simulink model "sampleModel1963_1"  (R2023a)
settings: Solver=VariableStepAuto  StartTime=0.0  StopTime=10.0  RelTol=1e-3
libraries: hdlsllib x5
settings Model: Creator=user1  LastModifiedBy=user1

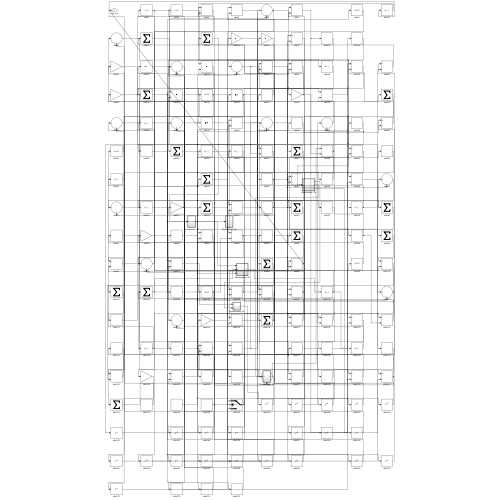
[thumbnail: Simulink's stored preview of the top-level diagram]
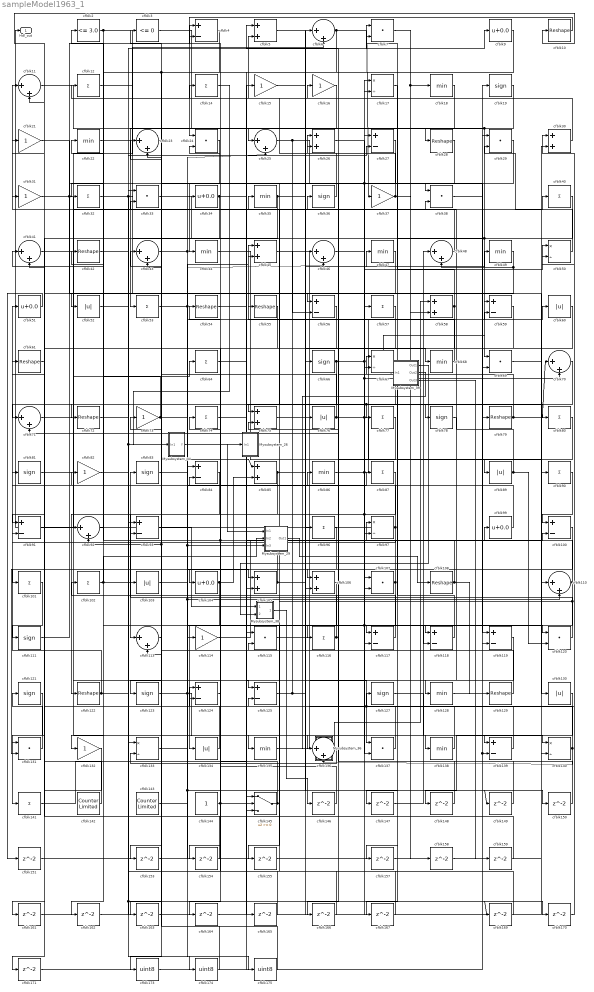
== system sampleModel1963_1 ==
  Mysubsystem_26 : Subsystem  TreatAsAtomicUnit=on  RTWFcnName=Mysubsystem_26
      settings: RTWFcnNameOpts=User specified  RTWFileNameOpts=Use function name
  Mysubsystem_29 : Subsystem  TreatAsAtomicUnit=on  RTWFcnName=Mysubsystem_29
      settings: RTWFcnNameOpts=User specified  RTWFileNameOpts=Use function name
  Mysubsystem_34 : Subsystem  TreatAsAtomicUnit=on  RTWFcnName=Mysubsystem_34
      settings: RTWFcnNameOpts=User specified  RTWFileNameOpts=Use function name
  Mysubsystem_36 : Subsystem  TreatAsAtomicUnit=on  RTWFcnName=Mysubsystem_36
      settings: RTWFcnNameOpts=User specified  RTWFileNameOpts=Use function name
  Mysubsystem_38 : Subsystem  TreatAsAtomicUnit=on  RTWFcnName=Mysubsystem_38
      settings: RTWFcnNameOpts=User specified  RTWFileNameOpts=Use function name
  Mysubsystem_39 : Subsystem  TreatAsAtomicUnit=on  RTWFcnName=Mysubsystem_39
      settings: RTWFcnNameOpts=User specified  RTWFileNameOpts=Use function name
  cfblk{10,28,42,54..55,61,72,79,108,122,129} (11 alike) : Reshape
  cfblk{4,27,56,59,84,91,93,100,117..119,124..125,139} (14 alike) : Sum  Inputs=+-  OutDataTypeStr=uint8
  cfblk{12,14,32,40,53,57,64,74,77,80,87,90,96,101..102,116,141} (17 alike) : Sum  Inputs=+  OutDataTypeStr=uint8
  cfblk{52,60,76,89,103,130,134} (7 alike) : Abs  OutDataTypeStr=uint8  SaturateOnIntegerOverflow=off
  cfblk{9,34,51,99,104} (5 alike) : Bias  Bias=0.0  SaturateOnIntegerOverflow=off
  cfblk{5,26,30,45,58,75,85,105..106} (9 alike) : Sum  OutDataTypeStr=uint8
  cfblk{7,24,29,33,38,69,107,115,120,131,137} (11 alike) : DotProduct  OutDataTypeStr=uint8
  cfblk{6,11,23,25,41,43,46,48,70..71,92,110,113,136} (14 alike) : Sum  Inputs=|++  OutDataTypeStr=uint8
  cfblk{19,36,66,78,81,83,111,121,123,127} (10 alike) : Signum
  cfblk{15..16,21,31,37,73,82,114,132} (9 alike) : Gain  OutDataTypeStr=uint8
  cfblk{18,22,35,44,47,49,68,86,128,135,138} (11 alike) : MinMax  OutDataTypeStr=uint8
  cfblk{17,50,67,97,133,140} (6 alike) : Product  Inputs=*/  OutDataTypeStr=uint8  RndMeth=Zero  SaturateOnIntegerOverflow=on
  cfblk142 : hdlsllib/Sources/Counter Limited  uplimit=7  tsamp=-1
  cfblk143 : hdlsllib/Sources/Counter Limited  uplimit=7  tsamp=-1
  cfblk144 : Constant  OutDataTypeStr=uint8  SampleTime=-1
  cfblk145 : Switch  OutDataTypeStr=uint8  SaturateOnIntegerOverflow=off  InputSameDT=off
  cfblk{146..151,153..155,157..159,161..167,169..171} (22 alike) : Delay  SampleTime=1
  cfblk173 : DataTypeConversion  OutDataTypeStr=uint8  SaturateOnIntegerOverflow=off  RndMeth=Floor
  cfblk174 : DataTypeConversion  OutDataTypeStr=uint8  SaturateOnIntegerOverflow=off  RndMeth=Floor
  cfblk175 : DataTypeConversion  OutDataTypeStr=uint8  SaturateOnIntegerOverflow=off  RndMeth=Floor
  cfblk2 : hdlsllib/Logic and Bit Operations/Compare To Constant  relop=<=  const=3.0  OutDataTypeStr=uint8
  cfblk3 : hdlsllib/Logic and Bit Operations/Compare To Zero  relop=<=  OutDataTypeStr=uint8
  Hdl_out : Outport  OutDataTypeStr=uint8
  wires:
  cfblk81/1 -> cfblk139/1
  cfblk110/1 -> cfblk117/2, cfblk163/1, cfblk3/1
  cfblk92/1 -> cfblk22/1
  cfblk108/1 -> cfblk129/1, cfblk26/2
  cfblk104/1 -> cfblk134/1, cfblk85/2
  cfblk44/1 -> cfblk89/1
  cfblk10/1 -> cfblk24/1
  cfblk115/1 -> cfblk30/1
  cfblk9/1 -> cfblk92/1, cfblk153/1
  cfblk121/1 -> cfblk141/1
  cfblk80/1 -> cfblk117/1
  cfblk45/1 -> cfblk137/1
  cfblk120/1 -> cfblk83/1, cfblk35/1
  cfblk137/1 -> cfblk127/1, cfblk41/2
  cfblk86/1 -> cfblk60/1, cfblk118/2
  cfblk16/1 -> cfblk53/1
  cfblk122/1 -> cfblk51/1, cfblk40/1
  cfblk32/1 -> cfblk110/1, cfblk136/1
  cfblk61/1 -> cfblk10/1
  cfblk3/1 -> cfblk69/1
  cfblk23/1 -> cfblk173/1
  cfblk124/1 -> cfblk54/1
  cfblk28/1 -> cfblk67/2, cfblk166/1
  cfblk101/1 -> cfblk111/1
  cfblk47/1 -> cfblk71/1
  cfblk71/1 -> cfblk36/1
  cfblk142/1 -> cfblk81/1
  cfblk34/1 -> cfblk91/1, cfblk170/1
  cfblk48/1 -> cfblk11/1
  cfblk107/1 -> cfblk74/1, cfblk41/1, cfblk155/1
  cfblk37/1 -> cfblk14/1, cfblk58/2
  cfblk114/1 -> cfblk97/1
  cfblk140/1 -> cfblk43/1, cfblk136/2
  cfblk24/1 -> cfblk44/1
  cfblk82/1 -> cfblk27/2, Mysubsystem_26/1(In1)
  cfblk79/1 -> cfblk70/1, cfblk16/1
  cfblk57/1 -> cfblk104/1
  cfblk40/1 -> cfblk59/1, cfblk167/1
  cfblk19/1 -> Mysubsystem_39/1(In1), cfblk106/2
  cfblk38/1 -> cfblk19/1
  cfblk138/1 -> cfblk26/1
  cfblk83/1 -> cfblk59/2
  cfblk31/1 -> cfblk125/1, cfblk34/1
  cfblk105/1 -> cfblk2/1, cfblk7/2
  cfblk87/1 -> cfblk97/2, cfblk164/1
  cfblk11/1 -> cfblk76/1
  cfblk78/1 -> cfblk128/1
  cfblk30/1 -> cfblk5/2
  cfblk22/1 -> cfblk96/1
  cfblk131/1 -> cfblk121/1
  cfblk69/1 -> cfblk90/1
  cfblk29/1 -> cfblk75/1
  cfblk123/1 -> cfblk138/1, cfblk45/2
  cfblk58/1 -> cfblk7/1, cfblk157/1
  cfblk91/1 -> cfblk64/1
  cfblk84/1 -> cfblk122/1
  cfblk18/1 -> cfblk25/1
  cfblk67/1 -> cfblk131/1
  cfblk106/1 -> cfblk132/1
  cfblk113/1 -> cfblk73/1
  cfblk103/1 -> cfblk149/1, cfblk175/1
  cfblk59/1 -> cfblk107/2
  cfblk119/1 -> cfblk145/2
  cfblk133/1 -> cfblk87/1
  cfblk5/1 -> cfblk66/1
  cfblk145/1 -> cfblk124/1, cfblk55/1
  cfblk75/1 -> cfblk49/1
  cfblk54/1 -> cfblk115/1
  cfblk141/1 -> cfblk15/1
  cfblk25/1 -> cfblk38/1, cfblk56/2
  cfblk134/1 -> cfblk61/1
  cfblk85/1 -> cfblk113/1, cfblk118/1
  cfblk90/1 -> cfblk100/1
  cfblk41/1 -> cfblk6/2
  cfblk144/1 -> cfblk24/2, cfblk99/1
  cfblk128/1 -> cfblk100/2
  cfblk111/1 -> cfblk4/1
  cfblk117/1 -> cfblk102/1
  cfblk42/1 -> cfblk103/1
  cfblk74/1 -> cfblk80/1
  cfblk33/1 -> cfblk119/1
  cfblk6/1 -> cfblk37/1, cfblk105/2
  cfblk127/1 -> cfblk140/1
  cfblk43/1 -> cfblk135/1, Mysubsystem_29/3(In3), cfblk25/2
  cfblk49/1 -> cfblk48/2, cfblk123/1
  cfblk143/1 -> cfblk114/1
  cfblk27/1 -> cfblk113/2
  cfblk4/1 -> cfblk52/1
  cfblk7/1 -> cfblk18/1, cfblk158/1
  cfblk46/1 -> cfblk17/1
  cfblk118/1 -> cfblk67/1
  cfblk36/1 -> cfblk12/1
  cfblk12/1 -> cfblk79/1
  cfblk89/1 -> cfblk38/2, cfblk120/2
  cfblk66/1 -> cfblk78/1, cfblk70/2, cfblk50/1, cfblk72/1
  cfblk73/1 -> cfblk42/1, cfblk105/1
  cfblk2/1 -> cfblk32/1, cfblk28/1
  cfblk53/1 -> cfblk120/1, cfblk110/2, cfblk85/1, cfblk46/2
  cfblk129/1 -> cfblk33/2, cfblk92/2
  cfblk76/1 -> cfblk17/2, cfblk130/1, cfblk31/1
  cfblk60/1 -> cfblk137/2
  cfblk50/1 -> cfblk29/2
  cfblk135/1 -> cfblk27/1
  cfblk35/1 -> cfblk101/1, cfblk68/1
  cfblk52/1 -> cfblk169/1, cfblk174/1
  cfblk72/1 -> cfblk93/1
  cfblk100/1 -> cfblk131/2
  cfblk21/1 -> cfblk56/1
  cfblk26/1 -> cfblk57/1
  cfblk70/1 -> cfblk116/1, cfblk77/1
  cfblk136/1 -> cfblk133/2
  cfblk77/1 -> cfblk106/1
  cfblk139/1 -> cfblk84/2
  cfblk102/1 -> Mysubsystem_29/2(In2), cfblk9/1
  cfblk125/1 -> cfblk47/1, cfblk46/1
  cfblk116/1 -> cfblk86/1, cfblk93/2
  cfblk99/1 -> cfblk82/1
  cfblk68/1 -> cfblk45/1
  cfblk97/1 -> cfblk91/2, cfblk21/1, Hdl_out/1
  cfblk146/1 -> cfblk124/2
  cfblk17/1 -> cfblk147/1
  cfblk147/1 -> cfblk48/1
  cfblk130/1 -> cfblk148/1
  cfblk148/1 -> cfblk5/1
  cfblk149/1 -> cfblk75/2
  cfblk15/1 -> cfblk150/1
  cfblk150/1 -> cfblk71/2
  cfblk51/1 -> cfblk151/1
  cfblk151/1 -> cfblk140/2
  cfblk153/1 -> cfblk84/1
  cfblk96/1 -> cfblk154/1
  cfblk154/1 -> cfblk43/2
  cfblk155/1 -> cfblk125/2
  cfblk157/1 -> cfblk29/1
  cfblk158/1 -> cfblk119/2
  cfblk159/1 -> cfblk11/2
  cfblk132/1 -> cfblk161/1
  cfblk161/1 -> cfblk30/2
  cfblk56/1 -> cfblk162/1
  cfblk162/1 -> cfblk33/1
  cfblk163/1 -> cfblk107/1
  cfblk164/1 -> cfblk6/1
  cfblk64/1 -> cfblk165/1
  cfblk165/1 -> cfblk133/1
  cfblk166/1 -> cfblk145/1
  cfblk167/1 -> cfblk115/2
  cfblk169/1 -> cfblk4/2
  cfblk170/1 -> cfblk50/2
  cfblk55/1 -> cfblk171/1
  cfblk171/1 -> cfblk145/3
  cfblk173/1 -> cfblk139/2, cfblk69/2
  cfblk174/1 -> cfblk23/1
  cfblk175/1 -> cfblk23/2
  Mysubsystem_29/1(Out1) -> cfblk108/1
  cfblk14/1 -> Mysubsystem_34/1(In1)
  Mysubsystem_34/1(Y) -> Mysubsystem_29/1(In1)
  Mysubsystem_36/1(Out1) -> cfblk58/1
  cfblk93/1 -> Mysubsystem_38/1(In1)
  Mysubsystem_38/1(Out1) -> cfblk146/1
  Mysubsystem_39/1(Out1) -> Mysubsystem_38/2(In2)
  Mysubsystem_39/2(Out2) -> Mysubsystem_36/1(In1)
  Mysubsystem_39/3(Out3) -> cfblk159/1

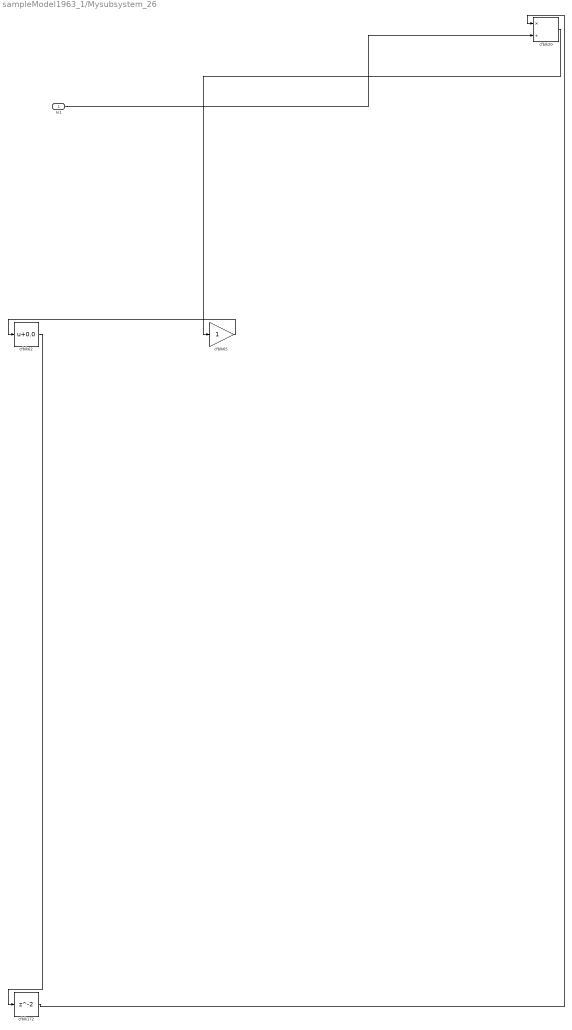
== system sampleModel1963_1/Mysubsystem_26 ==
  In1 : Inport
  cfblk172 : Delay  SampleTime=1
  cfblk20 : Product  Inputs=*/  RndMeth=Zero  SaturateOnIntegerOverflow=on
  cfblk62 : Bias  Bias=0.0  SaturateOnIntegerOverflow=off
  cfblk65 : Gain
  wires:
  cfblk65/1 -> cfblk62/1
  cfblk62/1 -> cfblk172/1
  cfblk172/1 -> cfblk20/1
  In1/1 -> cfblk20/2
  cfblk20/1 -> cfblk65/1

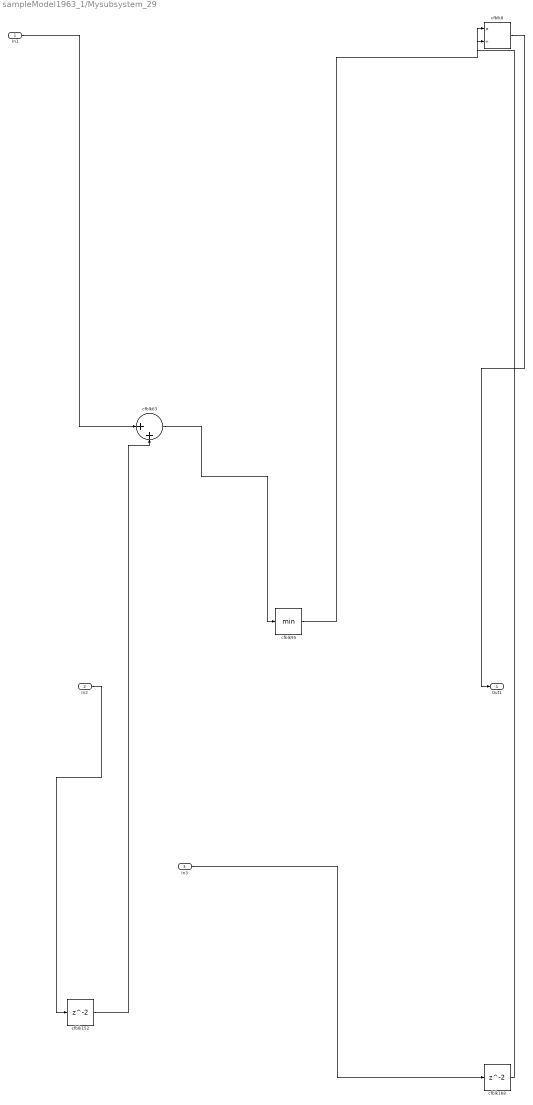
== system sampleModel1963_1/Mysubsystem_29 ==
  In1 : Inport
  In2 : Inport  Port=2
  In3 : Inport  Port=3
  cfblk152 : Delay  SampleTime=1
  cfblk168 : Delay  SampleTime=1
  cfblk63 : Sum  Inputs=|++
  cfblk8 : Product  Inputs=*/  RndMeth=Zero  SaturateOnIntegerOverflow=on
  cfblk95 : MinMax
  Out1 : Outport
  wires:
  In2/1 -> cfblk152/1
  cfblk8/1 -> Out1/1
  cfblk95/1 -> cfblk8/1
  cfblk152/1 -> cfblk63/2
  cfblk168/1 -> cfblk8/2
  cfblk63/1 -> cfblk95/1
  In1/1 -> cfblk63/1
  In3/1 -> cfblk168/1

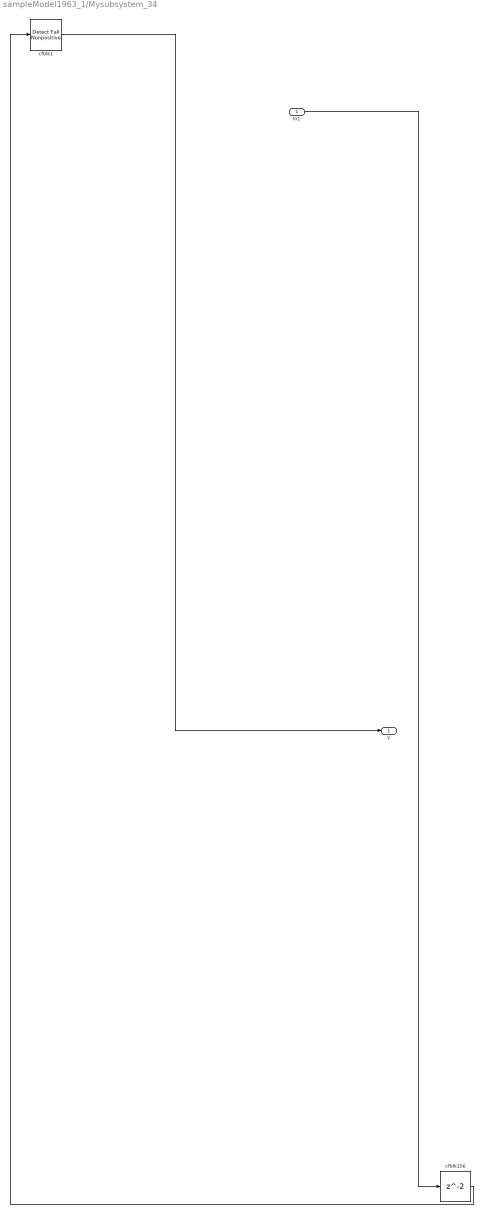
== system sampleModel1963_1/Mysubsystem_34 ==
  In1 : Inport
  cfblk1 : hdlsllib/Logic and Bit Operations/Detect Fall Nonpositive  vinit=0  OutDataTypeStr=boolean
  cfblk156 : Delay  SampleTime=1
  Y : Outport
  wires:
  cfblk156/1 -> cfblk1/1
  cfblk1/1 -> Y/1
  In1/1 -> cfblk156/1

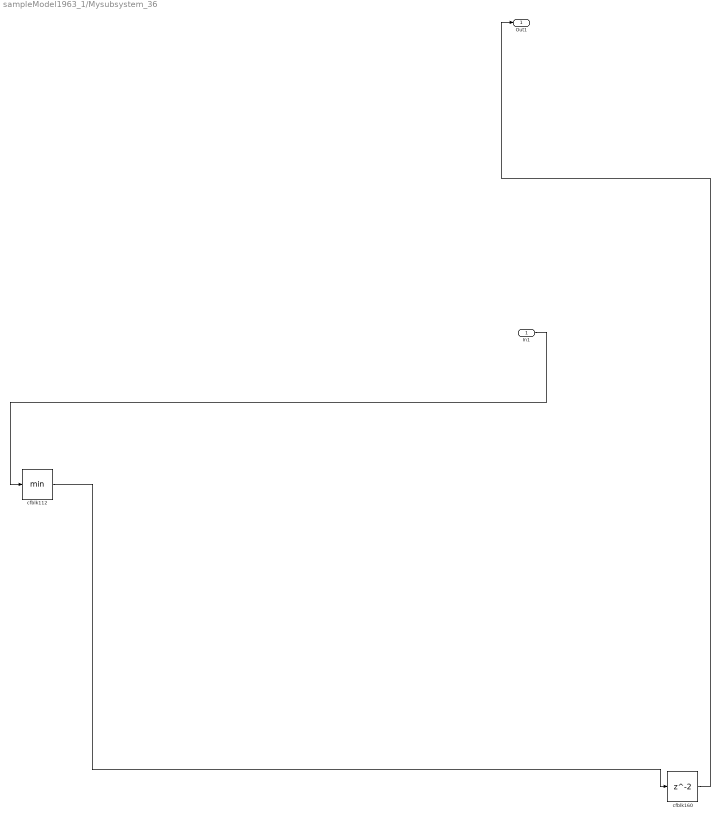
== system sampleModel1963_1/Mysubsystem_36 ==
  In1 : Inport
  cfblk112 : MinMax
  cfblk160 : Delay  SampleTime=1
  Out1 : Outport
  wires:
  cfblk112/1 -> cfblk160/1
  In1/1 -> cfblk112/1
  cfblk160/1 -> Out1/1

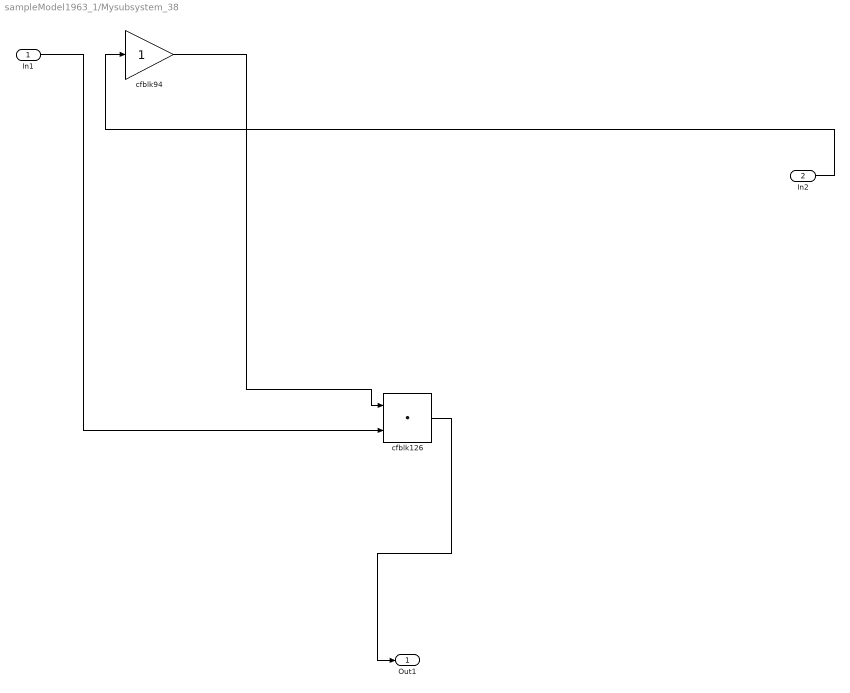
== system sampleModel1963_1/Mysubsystem_38 ==
  In1 : Inport
  In2 : Inport  Port=2
  cfblk126 : DotProduct  OutDataTypeStr=Inherit: Inherit via internal rule
  cfblk94 : Gain
  Out1 : Outport
  wires:
  cfblk94/1 -> cfblk126/1
  In1/1 -> cfblk126/2
  cfblk126/1 -> Out1/1
  In2/1 -> cfblk94/1

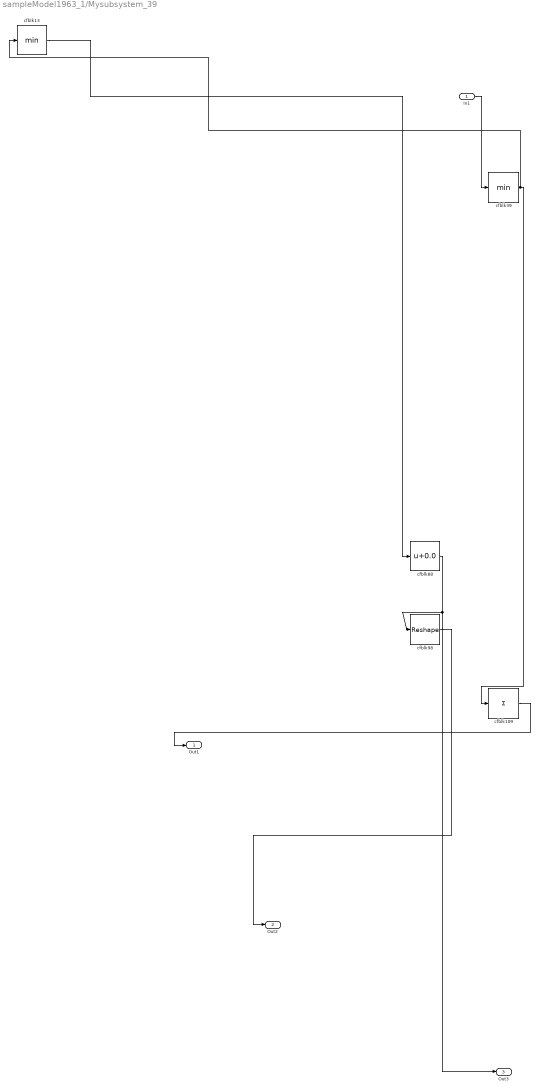
== system sampleModel1963_1/Mysubsystem_39 ==
  In1 : Inport
  cfblk109 : Sum  Inputs=+
  cfblk13 : MinMax
  cfblk39 : MinMax
  cfblk88 : Bias  Bias=0.0  SaturateOnIntegerOverflow=off
  cfblk98 : Reshape
  Out1 : Outport
  Out2 : Outport  Port=2
  Out3 : Outport  Port=3
  wires:
  cfblk109/1 -> Out1/1
  cfblk39/1 -> cfblk109/1, cfblk13/1
  cfblk88/1 -> Out3/1, cfblk98/1
  cfblk13/1 -> cfblk88/1
  cfblk98/1 -> Out2/1
  In1/1 -> cfblk39/1
